simulink model "modelo_completo_apresentado"  (R2017b)
settings: Solver=VariableStepAuto  StartTime=0.0  StopTime=5  RelTol=1e-3
libraries: simulink x5
settings Model: Creator=jorgeluis  LastModifiedBy=jorgeluis

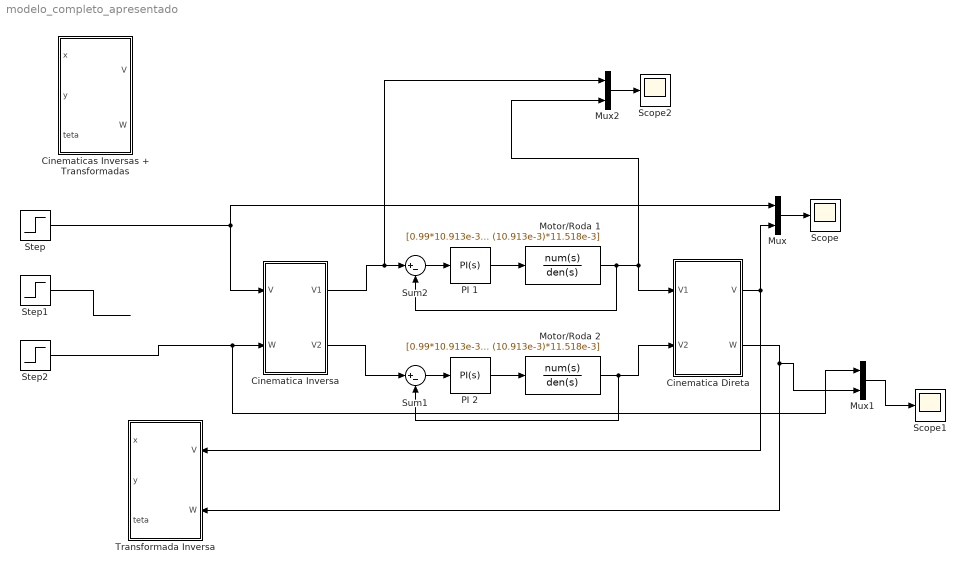
== system modelo_completo_apresentado ==
  Cinematica Direta : Subsystem
  Cinematica Inversa : Subsystem
  Cinematicas Inversas + Transformadas : Subsystem
  Motor/Roda 1 : TransferFcn  Numerator=[0.99*10.913e-3]  Denominator=[(1.5506*9.35604e-3) (10.913e-3)*11.518e-3]
  Motor/Roda 2 : TransferFcn  Numerator=[0.99*10.913e-3]  Denominator=[(1.5506*9.35604e-3) (10.913e-3)*11.518e-3]
  Mux : Mux  Inputs=2
  Mux1 : Mux  Inputs=2
  Mux2 : Mux  Inputs=2
  PI 1 : simulink/Continuous/PID Controller  Controller=PI  TimeDomain=Continuous-time  SampleTime=-1  IntegratorMethod=Forward Euler  FilterMethod=Forward Euler  Form=Ideal  UseFilter=on  ControllerParametersSource=internal  P=1.0800  I=0.0433  D=0  N=0  InitialConditionSource=internal  InitialConditionForIntegrator=0  InitialConditionForFilter=0  ExternalReset=none  LimitOutput=off  UpperSaturationLimit=inf  LowerSaturationLimit=-inf  LinearizeAsGain=on  AntiWindupMode=none  Kb=1  TrackingMode=off  Kt=1  PParamMin=[]  PParamMax=[]  IParamMin=[]  IParamMax=[]  DParamMin=[]  DParamMax=[]  NParamMin=[]  NParamMax=[]  KbParamMin=[]  KbParamMax=[]  KtParamMin=[]  KtParamMax=[]  POutMin=[]  POutMax=[]  IOutMin=[]  IOutMax=[]  DOutMin=[]  DOutMax=[]  NOutMin=[]  NOutMax=[]  KbOutMin=[]  KbOutMax=[]  KtOutMin=[]  KtOutMax=[]  IntegratorOutMin=[]  IntegratorOutMax=[]  FilterOutMin=[]  FilterOutMax=[]  SumOutMin=[]  SumOutMax=[]  SumI1OutMin=[]  SumI1OutMax=[]  SumI2OutMin=[]  SumI2OutMax=[]  SumI3OutMin=[]  SumI3OutMax=[]  SumDOutMin=[]  SumDOutMax=[]  SaturationOutMin=[]  SaturationOutMax=[]  IntegratorContinuousStateAttributes=''  IntegratorStateMustResolveToSignalObject=off  IntegratorRTWStateStorageClass=Auto  FilterContinuousStateAttributes=''  FilterStateMustResolveToSignalObject=off  FilterRTWStateStorageClass=Auto  DifferentiatorICPrevScaledInput=0  DifferentiatorOutMin=[]  DifferentiatorOutMax=[]  InitialConditionSetting=State (most efficient)  FilterDiffOutCoefMin=[]  FilterDiffOutCoefMax=[]  SumDenOutMin=[]  SumDenOutMax=[]  SumNumOutMin=[]  SumNumOutMax=[]  ReciprocalOutMin=[]  ReciprocalOutMax=[]  DivideOutMin=[]  DivideOutMax=[]  TunerSelectOption=Transfer Function Based (PID Tuner App)
  PI 2 : simulink/Continuous/PID Controller  Controller=PI  TimeDomain=Continuous-time  SampleTime=-1  IntegratorMethod=Forward Euler  FilterMethod=Forward Euler  Form=Ideal  UseFilter=on  ControllerParametersSource=internal  P=1.0800  I=0.0433  D=0  N=0  InitialConditionSource=internal  InitialConditionForIntegrator=0  InitialConditionForFilter=0  ExternalReset=none  LimitOutput=off  UpperSaturationLimit=inf  LowerSaturationLimit=-inf  LinearizeAsGain=on  AntiWindupMode=none  Kb=1  TrackingMode=off  Kt=1  PParamMin=[]  PParamMax=[]  IParamMin=[]  IParamMax=[]  DParamMin=[]  DParamMax=[]  NParamMin=[]  NParamMax=[]  KbParamMin=[]  KbParamMax=[]  KtParamMin=[]  KtParamMax=[]  POutMin=[]  POutMax=[]  IOutMin=[]  IOutMax=[]  DOutMin=[]  DOutMax=[]  NOutMin=[]  NOutMax=[]  KbOutMin=[]  KbOutMax=[]  KtOutMin=[]  KtOutMax=[]  IntegratorOutMin=[]  IntegratorOutMax=[]  FilterOutMin=[]  FilterOutMax=[]  SumOutMin=[]  SumOutMax=[]  SumI1OutMin=[]  SumI1OutMax=[]  SumI2OutMin=[]  SumI2OutMax=[]  SumI3OutMin=[]  SumI3OutMax=[]  SumDOutMin=[]  SumDOutMax=[]  SaturationOutMin=[]  SaturationOutMax=[]  IntegratorContinuousStateAttributes=''  IntegratorStateMustResolveToSignalObject=off  IntegratorRTWStateStorageClass=Auto  FilterContinuousStateAttributes=''  FilterStateMustResolveToSignalObject=off  FilterRTWStateStorageClass=Auto  DifferentiatorICPrevScaledInput=0  DifferentiatorOutMin=[]  DifferentiatorOutMax=[]  InitialConditionSetting=State (most efficient)  FilterDiffOutCoefMin=[]  FilterDiffOutCoefMax=[]  SumDenOutMin=[]  SumDenOutMax=[]  SumNumOutMin=[]  SumNumOutMax=[]  ReciprocalOutMin=[]  ReciprocalOutMax=[]  DivideOutMin=[]  DivideOutMax=[]  TunerSelectOption=Transfer Function Based (PID Tuner App)
  Scope : Scope
  Scope1 : Scope
  Scope2 : Scope
  Step : Step  Time=0  After=5  SampleTime=0
  Step1 : Step  Time=0  After=3  SampleTime=0
  Step2 : Step  Time=0  After=1.5  SampleTime=0
  Sum1 : Sum  Inputs=|+-
  Sum2 : Sum  Inputs=|+-
  Transformada Inversa : Subsystem
  wires:
  Sum1/1 -> PI 2/1
  PI 2/1 -> Motor/Roda 2/1
  PI 1/1 -> Motor/Roda 1/1
  Sum2/1 -> PI 1/1
  Cinematica Inversa/1(V1) -> Mux2/1, Sum2/1
  Cinematica Inversa/2(V2) -> Sum1/1
  Motor/Roda 1/1 -> Sum2/2, Cinematica Direta/1(V1), Mux2/2
  Motor/Roda 2/1 -> Sum1/2, Cinematica Direta/2(V2)
  Cinematica Direta/1(V) -> Mux/2, Transformada Inversa/1(V)
  Cinematica Direta/2(W) -> Mux1/2, Transformada Inversa/2(W)
  Step/1 -> Cinematica Inversa/1(V), Mux/1
  Step2/1 -> Mux1/1, Cinematica Inversa/2(W)
  Step1/1 -> ?
  Mux/1 -> Scope/1
  Mux1/1 -> Scope1/1
  Mux2/1 -> Scope2/1

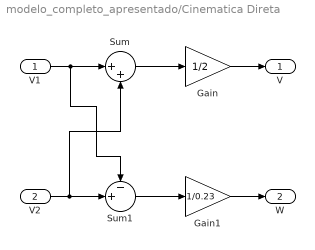
== system modelo_completo_apresentado/Cinematica Direta ==
  V1 : Inport
  V2 : Inport  Port=2
  Gain : Gain  Gain=1/2
  Gain1 : Gain  Gain=1/0.23
  Sum : Sum  Inputs=|++
  Sum1 : Sum  Inputs=-+|
  V : Outport
  W : Outport  Port=2
  wires:
  V2/1 -> Sum/2, Sum1/2
  V1/1 -> Sum1/1, Sum/1
  Sum/1 -> Gain/1
  Gain1/1 -> W/1
  Gain/1 -> V/1
  Sum1/1 -> Gain1/1

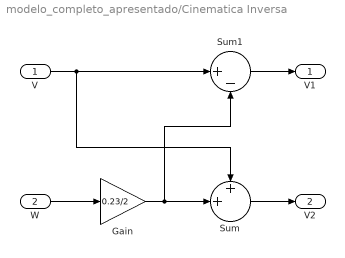
== system modelo_completo_apresentado/Cinematica Inversa ==
  V : Inport
  W : Inport  Port=2
  Gain : Gain  Gain=0.23/2
  Sum : Sum  Inputs=++|
  Sum1 : Sum  Inputs=|+-
  V1 : Outport
  V2 : Outport  Port=2
  wires:
  W/1 -> Gain/1
  Sum1/1 -> V1/1
  Gain/1 -> Sum1/2, Sum/2
  V/1 -> Sum/1, Sum1/1
  Sum/1 -> V2/1

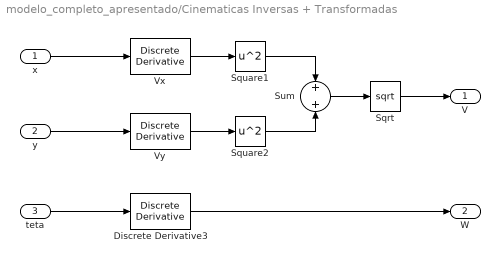
== system modelo_completo_apresentado/Cinematicas Inversas + Transformadas ==
  x : Inport
  y : Inport  Port=2
  teta : Inport  Port=3
  Discrete Derivative3 : simulink/Discrete/Discrete Derivative  gainval=1.0  ICPrevScaledInput=0.0  OutMin=[]  OutMax=[]  OutDataType=fixdt(1, 16)  OutScaling=2^-10  DoSatur=off
  Sqrt : Sqrt  SaturateOnIntegerOverflow=on
  Square1 : Math  Operator=square  RndMeth=Zero  SaturateOnIntegerOverflow=on
  Square2 : Math  Operator=square  RndMeth=Zero  SaturateOnIntegerOverflow=on
  Sum : Sum  Inputs=+|+
  Vx : simulink/Discrete/Discrete Derivative  gainval=1.0  ICPrevScaledInput=0.0  OutMin=[]  OutMax=[]  OutDataType=fixdt(1, 16)  OutScaling=2^-10  DoSatur=off
  Vy : simulink/Discrete/Discrete Derivative  gainval=1.0  ICPrevScaledInput=0.0  OutMin=[]  OutMax=[]  OutDataType=fixdt(1, 16)  OutScaling=2^-10  DoSatur=off
  V : Outport
  W : Outport  Port=2
  wires:
  Discrete Derivative3/1 -> W/1
  teta/1 -> Discrete Derivative3/1
  x/1 -> Vx/1
  Sqrt/1 -> V/1
  y/1 -> Vy/1
  Vx/1 -> Square1/1
  Vy/1 -> Square2/1
  Square1/1 -> Sum/1
  Square2/1 -> Sum/2
  Sum/1 -> Sqrt/1

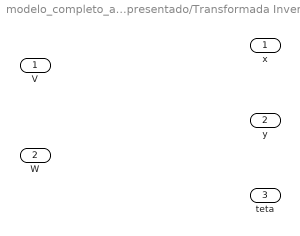
== system modelo_completo_apresentado/Transformada Inversa ==
  V : Inport
  W : Inport  Port=2
  x : Outport
  y : Outport  Port=2
  teta : Outport  Port=3
